simulink model "kre_external_observer_wrapper"  (R2026a)
settings: Solver=FixedStepDiscrete  FixedStep=5e-5
settings Model: Creator=hzldx  LastModifiedBy=ASUS
settings HardwareCC: ProdLargestAtomicInteger=Long  ProdLargestAtomicFloat=Double  ProdHWDeviceType=ARM Compatible->ARM Cortex-M  TargetLargestAtomicInteger=Long  TargetLargestAtomicFloat=Double  TargetIntDivRoundTo=Zero  TargetEndianess=LittleEndian  TargetHWDeviceType=ARM Compatible->ARM Cortex-M  ProdEqTarget=off
settings RTWCC: SystemTargetFile=ert.tlc  GenCodeOnly=on  GenerateMakefile=off  Description=Embedded Coder
settings ERTTargetCC: GenerateSampleERTMain=on

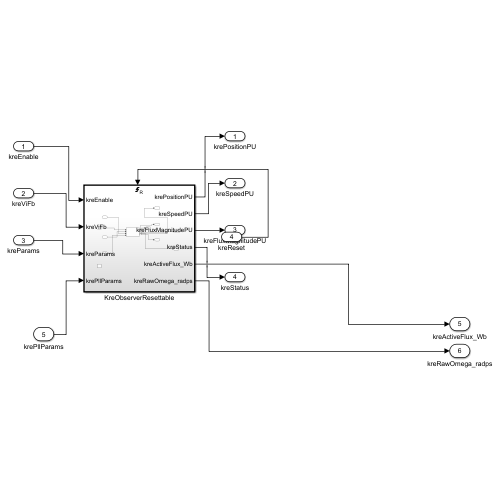
[thumbnail: Simulink's stored preview of the top-level diagram]
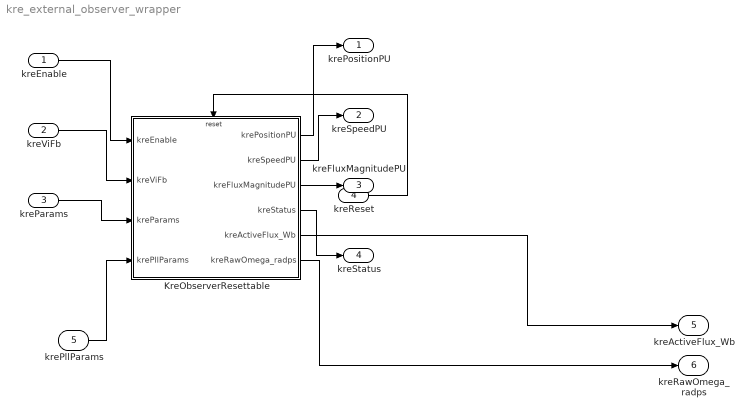
== system kre_external_observer_wrapper ==
  kreEnable : Inport  OutDataTypeStr=uint8  PortDimensions=1  SampleTime=5e-5
  kreViFb : Inport  Port=2  OutDataTypeStr=single  PortDimensions=[4 1]  SampleTime=5e-5
  kreParams : Inport  Port=3  OutDataTypeStr=single  PortDimensions=[14 1]  SampleTime=5e-5
  kreReset : Inport  Port=4  OutDataTypeStr=uint8  PortDimensions=1  SampleTime=5e-5
  krePllParams : Inport  Port=5  OutDataTypeStr=single  PortDimensions=[2 1]  SampleTime=5e-5
  KreObserverResettable : Subsystem  TreatAsAtomicUnit=on
  krePositionPU : Outport  OutDataTypeStr=single  PortDimensions=1  SampleTime=5e-5
  kreSpeedPU : Outport  Port=2  OutDataTypeStr=single  PortDimensions=1  SampleTime=5e-5
  kreFluxMagnitudePU : Outport  Port=3  OutDataTypeStr=single  PortDimensions=1  SampleTime=5e-5
  kreStatus : Outport  Port=4  OutDataTypeStr=uint8  PortDimensions=1  SampleTime=5e-5
  kreActiveFlux_Wb : Outport  Port=5
  kreRawOmega_radps : Outport  Port=6
  wires:
  KreObserverResettable/6(kreRawOmega_radps) -> kreRawOmega_radps/1
  KreObserverResettable/5(kreActiveFlux_Wb) -> kreActiveFlux_Wb/1
  krePllParams/1 -> KreObserverResettable/4(krePllParams)
  KreObserverResettable/4(kreStatus) -> kreStatus/1
  KreObserverResettable/3(kreFluxMagnitudePU) -> kreFluxMagnitudePU/1
  KreObserverResettable/2(kreSpeedPU) -> kreSpeedPU/1
  KreObserverResettable/1(krePositionPU) -> krePositionPU/1
  kreParams/1 -> KreObserverResettable/3(kreParams)
  kreViFb/1 -> KreObserverResettable/2(kreViFb)
  kreEnable/1 -> KreObserverResettable/1(kreEnable)
  kreReset/1 -> KreObserverResettable/Reset

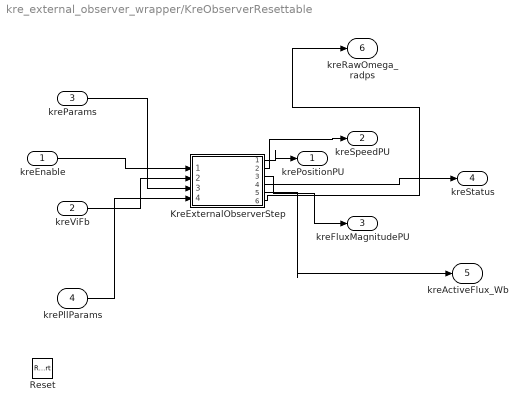
== system kre_external_observer_wrapper/KreObserverResettable ==
  kreEnable : Inport  OutDataTypeStr=uint8  PortDimensions=1  SampleTime=5e-5
  kreViFb : Inport  Port=2  OutDataTypeStr=single  PortDimensions=[4 1]  SampleTime=5e-5
  kreParams : Inport  Port=3  OutDataTypeStr=single  PortDimensions=[14 1]  SampleTime=5e-5
  krePllParams : Inport  Port=4  OutDataTypeStr=single  PortDimensions=[2 1]  SampleTime=5e-5
  Reset : ResetPort  DisableCoverage=on
  KreExternalObserverStep : MATLAB Function  TreatAsAtomicUnit=on
  krePositionPU : Outport  OutDataTypeStr=single  PortDimensions=1  SampleTime=5e-5
  kreSpeedPU : Outport  Port=2  OutDataTypeStr=single  PortDimensions=1  SampleTime=5e-5
  kreFluxMagnitudePU : Outport  Port=3  OutDataTypeStr=single  PortDimensions=1  SampleTime=5e-5
  kreStatus : Outport  Port=4  OutDataTypeStr=uint8  PortDimensions=1  SampleTime=5e-5
  kreActiveFlux_Wb : Outport  Port=5
  kreRawOmega_radps : Outport  Port=6
  wires:
  kreEnable/1 -> KreExternalObserverStep/1(kreEnable)
  KreExternalObserverStep/1(krePositionPU) -> krePositionPU/1
  KreExternalObserverStep/6(kreRawOmega_radps) -> kreRawOmega_radps/1
  KreExternalObserverStep/5(kreActiveFlux_Wb) -> kreActiveFlux_Wb/1
  KreExternalObserverStep/4(kreStatus) -> kreStatus/1
  KreExternalObserverStep/3(kreFluxMagnitudePU) -> kreFluxMagnitudePU/1
  KreExternalObserverStep/2(kreSpeedPU) -> kreSpeedPU/1
  krePllParams/1 -> KreExternalObserverStep/4(krePllParams)
  kreParams/1 -> KreExternalObserverStep/3(kreParams)
  kreViFb/1 -> KreExternalObserverStep/2(kreViFb)

== matlab function kre_external_observer_wrapper/KreObserverResettable/KreExternalObserverStep ==
  data: kreEnable input; krePositionPU output; kreViFb input; kreParams input; krePllParams input; kreSpeedPU output; kreFluxMagnitudePU output; kreStatus output; kreActiveFlux_Wb output; kreRawOmega_radps output
function [krePositionPU, kreSpeedPU, kreFluxMagnitudePU, kreStatus, kreActiveFlux_Wb, kreRawOmega_radps] = fcn(kreEnable, kreViFb, kreParams, krePllParams)
%#codegen
[krePositionPU, kreSpeedPU, kreFluxMagnitudePU, kreActiveFlux_Wb, kreRawOmega_radps, kreStatus] = kre_external_observer_diagnostic_step(kreEnable, kreViFb, kreParams, krePllParams);
end
